simulink model "suivi_ligne_huit_eleve_2022b"  (R2024b)
settings: Solver=VariableStepAuto  StartTime=0.0  StopTime=140  RelTol=1e-3
InitFcn:
  | close all;
libraries: mobileRoboticsLib x2, visionsources x2, dspvision x2, visionsinks x2
settings Model: PacingRate=100  Creator=Caroline Lelandais  LastModifiedBy=radam
settings SolverCC: AlgebraicLoopSolver=TrustRegion
settings OptimizationCC: ReuseModelBlockBuffer=off
settings DebuggingCC: UnconnectedInputMsg=warning  UnconnectedOutputMsg=warning  UnconnectedLineMsg=warning
settings ModelReferenceCC: EnableRefExpFcnMdlSchedulingChecks=on
settings RTWCC: GPUComputeCapability=3.5

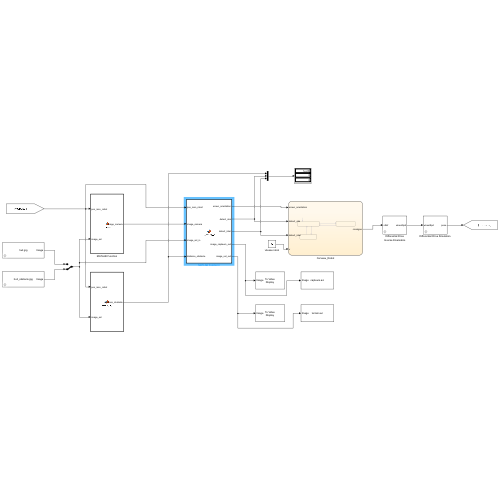
[thumbnail: Simulink's stored preview of the top-level diagram]
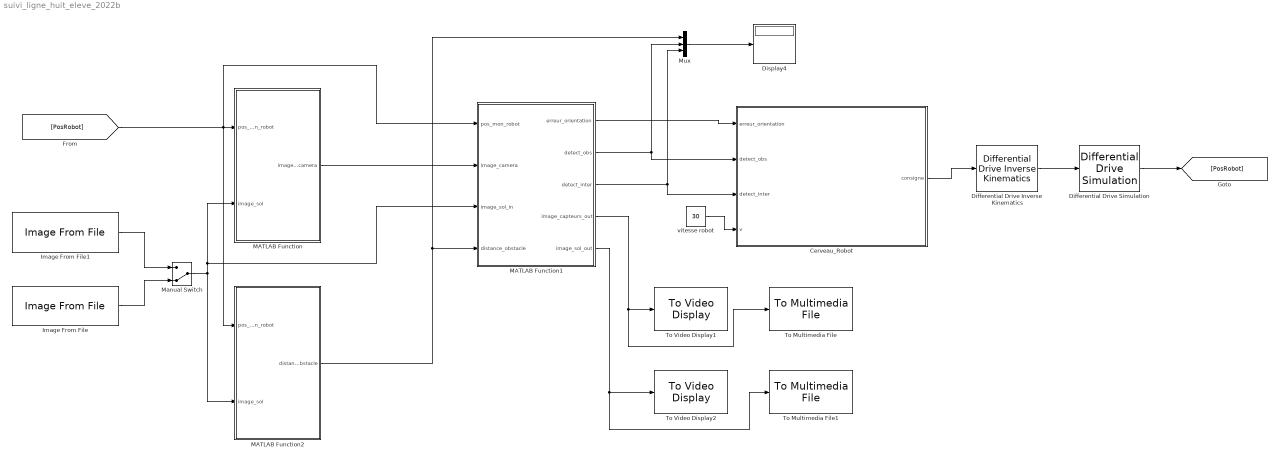
== system suivi_ligne_huit_eleve_2022b ==
  Cerveau_Robot : Stateflow chart  TreatAsAtomicUnit=on
  Differential Drive Inverse Kinematics : mobileRoboticsLib/Kinematic Models/Differential Drive/Differential Drive Inverse Kinematics  wheelRadius=0.1  wheelBase=0.5
      settings: SourceProductName=Mobile Robotics Simulation Toolbox
  Differential Drive Simulation : mobileRoboticsLib/Kinematic Models/Differential Drive/Differential Drive Simulation  wheelRadius=0.1  wheelBase=0.5  initX=291  initY=451  initAngle=2.4  Ts=0.1
      settings: SourceProductName=Mobile Robotics Simulation Toolbox
  Display4 : Display
  Image From File : visionsources/Image From File  Tag=vipblks_nd  FileName=huit_obstacle.jpg  Ts=inf  imagePorts=One multidimensional signal  OutPortLabels=R|G|B  ImageDataType=Inherit from input image  sdImageDataType=uint(8)  Signed=on  WordLength=16  FractionLengthMode=User-defined  FractionLength=15
  Image From File1 : visionsources/Image From File  Tag=vipblks_nd  FileName=huit.jpg  Ts=inf  imagePorts=One multidimensional signal  OutPortLabels=R|G|B  ImageDataType=Inherit from input image  sdImageDataType=uint(8)  Signed=on  WordLength=16  FractionLengthMode=User-defined  FractionLength=15
  MATLAB Function : MATLAB Function  TreatAsAtomicUnit=on
  MATLAB Function1 : MATLAB Function  TreatAsAtomicUnit=on
  MATLAB Function2 : MATLAB Function  TreatAsAtomicUnit=on
  Manual Switch : ManualSwitch  CurrentSetting=0
  Mux : Mux  Inputs=3
  To Multimedia File : dspvision/To Multimedia File  outputFilename=capteurs.avi  streamSelection=Video only  videoCompressor=None (uncompressed)  audioCompressor=None (uncompressed)  imagePorts=One multidimensional signal  fileType=AVI  audioDatatype=Determine from input data type  fourcc=RGB  audioBitRate=128  audioQuality=75  videoQuality=75  mj2000CompFactor=10
  To Multimedia File1 : dspvision/To Multimedia File  outputFilename=terrain.avi  streamSelection=Video only  videoCompressor=None (uncompressed)  audioCompressor=None (uncompressed)  imagePorts=One multidimensional signal  fileType=AVI  audioDatatype=Determine from input data type  fourcc=RGB  audioBitRate=128  audioQuality=75  videoQuality=75  mj2000CompFactor=10
  To Video Display1 : visionsinks/To Video Display  windowSizeMode=Normal  openAtMdlStart=on  fullScreen=off  videoWindowX=536805376  videoWindowY=536805376  saveWindowSize=off  videoWindowWidth=520  videoWindowHeight=352  inputColorFormat=RGB  inputType=Obsolete  imagePorts=One multidimensional signal  OutputDevice=On-screen video monitor  dataOrg=Column-major  isWindowOpen=off
  To Video Display2 : visionsinks/To Video Display  windowSizeMode=Normal  openAtMdlStart=on  fullScreen=off  videoWindowX=16  videoWindowY=88  saveWindowSize=off  videoWindowWidth=1247  videoWindowHeight=642  inputColorFormat=RGB  inputType=Obsolete  imagePorts=One multidimensional signal  OutputDevice=On-screen video monitor  dataOrg=Column-major  isWindowOpen=off
  vitesse robot : Constant  Value=30
  wires:
  Differential Drive Inverse Kinematics/1 -> Differential Drive Simulation/1
  Cerveau_Robot/1(consigne) -> Differential Drive Inverse Kinematics/1
  Differential Drive Simulation/1 -> [PosRobot]
  [PosRobot] -> MATLAB Function1/1(pos_mon_robot), MATLAB Function2/1(pos_mon_robot), MATLAB Function/1(pos_mon_robot)
  vitesse robot/1 -> Cerveau_Robot/4(v)
  MATLAB Function1/1(erreur_orientation) -> Cerveau_Robot/1(erreur_orientation)
  MATLAB Function1/2(detect_obs) -> Mux/2, Cerveau_Robot/2(detect_obs)
  MATLAB Function1/3(detect_inter) -> Mux/3, Cerveau_Robot/3(detect_inter)
  MATLAB Function1/4(image_capteurs_out) -> To Video Display1/1, To Multimedia File/1
  MATLAB Function1/5(image_sol_out) -> To Video Display2/1, To Multimedia File1/1
  MATLAB Function2/1(distance_obstacle) -> Mux/1, MATLAB Function1/4(distance_obstacle)
  MATLAB Function/1(image_camera) -> MATLAB Function1/2(image_camera)
  Manual Switch/1 -> MATLAB Function1/3(image_sol_in), MATLAB Function/2(image_sol), MATLAB Function2/2(image_sol)
  Image From File1/1 -> Manual Switch/1
  Image From File/1 -> Manual Switch/2
  Mux/1 -> Display4/1

== matlab function suivi_ligne_huit_eleve_2022b/MATLAB Function1 ==
  data: pos_mon_robot input; image_camera input; erreur_orientation output; detect_obs output; detect_inter output; image_sol_in input; image_capteurs_out output; image_sol_out output; distance_obstacle input
function [erreur_orientation, detect_obs, detect_inter, image_capteurs_out, image_sol_out] = Perception(pos_mon_robot, image_camera, image_sol_in, distance_obstacle)
%#codegen
% PERCEPTION (clean & simple, aligned with simplified Stateflow)
%   SuivreLigne : consigne = [v; erreur_orientation]
%   GererObs    : consigne = [0; +w_turn]  (handled in Stateflow)
%   GererInter  : consigne = [v; 0]        (handled in Stateflow)

% ---- init scalars ----
erreur_orientation = 0.0;  detect_obs = 0.0;  detect_inter = 0.0;

% ---- geometry ----
profondeur_camera=40; demi_largeur_camera=15;
profondeur_telemetre=80; demi_largeur_telemetre=5;
longueur_robot=30; demi_largeur_robot=10;

% ---- pose ----
px=round(pos_mon_robot(1)); py=round(pos_mon_robot(2)); th=pos_mon_robot(3);

% ---- memories ----
persistent ePrev obsLatch
if isempty(ePrev), ePrev=0; end
if isempty(obsLatch), obsLatch=0; end

% ---- outputs (fixed size) ----
image_capteurs_out=zeros(profondeur_telemetre,2*demi_largeur_camera,3,'uint8');
image_sol_out=image_sol_in; H=size(image_sol_out,1); W=size(image_sol_out,2);

% 1) LINE FOLLOWING — bottom 40% centroid on dark line
R=double(image_camera(:,:,1)); G=double(image_camera(:,:,2)); B=double(image_camera(:,:,3));
gray=0.2989*R+0.5870*G+0.1140*B;  Tdark=100;  isLine=(gray<Tdark);
rows=(profondeur_camera-round(0.4*profondeur_camera)+1):profondeur_camera; cols=1:(2*demi_largeur_camera);
colIdx=double(cols(:)); c0=demi_largeur_camera+0.5;
centers=nan(numel(rows),1);
for k=1:numel(rows)
    rr=rows(k); mask=isLine(rr,cols); n=nnz(mask);
    if n>0, centers(k)=sum(colIdx(mask))/n; end
end
Wrow=linspace(1,2,numel(rows))'; maskV=~isnan(centers);
cMean = c0; if any(maskV), cMean = sum(Wrow(maskV).*centers(maskV))/sum(Wrow(maskV)); end
offPix = c0 - cMean; offPix = max(-(demi_largeur_camera-3),min(demi_largeur_camera-3,offPix));
erreur_orientation = 0.6*ePrev + 0.4*offPix; ePrev=erreur_orientation;

% 2) OBSTACLE — simple distance with small hysteresis
dEnter=0.35*profondeur_telemetre; dExit=0.45*profondeur_telemetre;
d=double(distance_obstacle); if ~(isfinite(d))||d<=0||d>1e6, d=dExit+1; end
if obsLatch==0, if d<dEnter, obsLatch=1; end, else, if d>dExit, obsLatch=0; end, end
detect_obs=double(obsLatch);

% 3) INTERSECTION — white horizon test (only if no obstacle)
hRow=round(0.85*profondeur_camera); whiteCount=nnz(gray(hRow,:)>200);
detect_inter = double( (whiteCount/(2*demi_largeur_camera))>0.80 && detect_obs==0 );

% 4) VISUALS — same layout as before (camera, telemeter, overlays)
image_capteurs_out(1:profondeur_camera,1:2*demi_largeur_camera,:)=uint8(image_camera);
for i=(profondeur_camera+1):profondeur_telemetre
  for j=1:(2*demi_largeur_camera)
    c=(px+1j*py)+(i+1j*(j-demi_largeur_camera))*exp(1j*th);
    rr=min(max(1,round(real(c))),H); cc=min(max(1,round(imag(c))),W);
    image_capteurs_out(i,j,:)=image_sol_out(rr,cc,:);
  end
end
for i=1:longueur_robot
  for j=1:2*demi_largeur_robot
    c=(px+1j*py)-(i+1j*(j-demi_largeur_robot))*exp(1j*th);
    rr=min(max(1,round(real(c))),H); cc=min(max(1,round(imag(c))),W);
    image_sol_out(rr,cc,2)=255;
  end
end
for i=1:profondeur_camera
  for j=1:2*demi_largeur_camera
    c=(px+1j*py)+(i+1j*(j-demi_largeur_camera))*exp(1j*th);
    rr=min(max(1,round(real(c))),H); cc=min(max(1,round(imag(c))),W);
    image_sol_out(rr,cc,1)=255;
  end
end
for i=1:profondeur_telemetre
  for j=1:2*demi_largeur_telemetre
    c=(px+1j*py)+(i+1j*(j-demi_largeur_telemetre))*exp(1j*th);
    rr=min(max(1,round(real(c))),H); cc=min(max(1,round(imag(c))),W);
    image_sol_out(rr,cc,3)=255;
  end
end
pt=(px+1j*py)+(profondeur_camera/2+1j*erreur_orientation)*exp(1j*th);
r=min(max(1,round(real(pt))),H); c=min(max(1,round(imag(pt))),W);
image_sol_out(max(1,r-2):min(H,r+2),max(1,c-2):min(W,c+2),2)=255;
if abs(erreur_orientation)<(demi_largeur_camera-2)
  cc=round(demi_largeur_camera+0.5+erreur_orientation); lc=round(profondeur_camera/2);
  image_capteurs_out(max(1,lc-2):min(profondeur_camera,lc+2),max(1,cc-2):min(2*demi_largeur_camera,cc+2),2)=255;
end
image_capteurs_out(1,:,1)=240; image_capteurs_out(1:profondeur_camera,1,1)=240;
image_capteurs_out(profondeur_camera,:,1)=240; image_capteurs_out(1:profondeur_camera,end,1)=240;
k=(demi_largeur_camera-demi_largeur_telemetre);
image_capteurs_out(1,k:end-k,3)=240; image_capteurs_out(:,k,3)=240;
image_capteurs_out(end,k:end-k,3)=240; image_capteurs_out(:,end-k,3)=240;
image_capteurs_out=flipud(image_capteurs_out); image_capteurs_out=fliplr(image_capteurs_out);
image_sol_out(1:2,:,3)=240; image_sol_out(:,1:2,3)=240; image_sol_out(end-1:end,:,3)=240; image_sol_out(:,end-1:end,3)=240;
image_sol_out(px-1:px+1,py-1:py+1,2)=255;
end

== matlab function suivi_ligne_huit_eleve_2022b/MATLAB Function ==
  data: pos_mon_robot input; image_sol input; image_camera output
% Son rôle est de modéliser la photo brute prise par la caméra. Le modèle est extrêmement simplifié et fait comme si la photo était prise à la verticale et à l’avant du robot (par d’angle de vue).
% •	Entrées : pos_mon_robot (position du robot), image_sol (« terrain » soit la vue du ciel du circuit où doit évoluer le robot )
% •	Sorties : image_camera (vue du ciel du champ de vision du robot, rectangle rouge sur Video Display2)



function image_camera  = camera(pos_mon_robot, image_sol)

% Caractéristiques des coordonnées du champ de vision de la caméra 
profondeur_camera = 40;
demi_largeur_camera = 15;

% Récupération de la position du robot concerné
pos_x_vehicule = round(pos_mon_robot(1));
pos_y_vehicule = round(pos_mon_robot(2));
pos_angle_vehicule = pos_mon_robot(3);

%image vue par le capteur
image_camera=uint8(zeros(profondeur_camera,2*demi_largeur_camera,3));
for i=1:profondeur_camera
    for j=1:2*demi_largeur_camera
        c=(pos_x_vehicule+1j*pos_y_vehicule)+(i+1j*(j-demi_largeur_camera))*exp(1j*pos_angle_vehicule);
        image_camera(i,j,:)=image_sol(round(real(c)),round(imag(c)),:);
    end
end

== matlab function suivi_ligne_huit_eleve_2022b/MATLAB Function2 ==
  data: pos_mon_robot input; image_sol input; distance_obstacle output
% Son rôle est de modéliser le signal de sortie du télémètre à l’avant du robot.
% •	Entrées : pos_mon_robot (position du robot), image_sol (« terrain » soit la vue du ciel du circuit où doit évoluer le robot )
% •	Sorties : distance_obstacle (distance de l’obstacle)


function distance_obstacle    = telemetre(pos_mon_robot, image_sol)

% Caractéristiques des coordonnées du champ de vision du télémètre

profondeur_telemetre_x = 80;
largeur_telemetre_y = 5;

% Récupération de la position du robot concerné
pos_x_vehicule = round(pos_mon_robot(1));
pos_y_vehicule = round(pos_mon_robot(2));
pos_angle_vehicule = pos_mon_robot(3);

%image vue par le capteur et detection d'un obstacle
image_capteur2=uint8(zeros(profondeur_telemetre_x,2*largeur_telemetre_y,3));
distance_obstacle=100000;
for i=1:profondeur_telemetre_x
    for j=1:2*largeur_telemetre_y
        c=(pos_x_vehicule+1j*pos_y_vehicule)+(i+1j*(j-largeur_telemetre_y))*exp(1j*pos_angle_vehicule);
        image_capteur2(i,j,:)=image_sol(round(real(c)),round(imag(c)),:);
        if (image_capteur2(i,j,1)>200) && (image_capteur2(i,j,2)<50) && (image_capteur2(i,j,3)<50)   % obstacle simulé ici par couleur rouge
            distance_obstacle=min(distance_obstacle,abs((i+1j*j)-(0+1j*largeur_telemetre_y)));
        end
    end
end

== stateflow chart suivi_ligne_huit_eleve_2022b/Cerveau_Robot ==
  state SuivreLigne
    consigne = [v; erreur_orientation];
  state GererObs
    during: consigne=[0;+w]
  state GererInter
    during: consigne = [v; 0];
  (default) -> SuivreLigne
  SuivreLigne -> GererObs [order 1] : [detect_obs == 1]
  GererObs -> SuivreLigne : [after(pi/w, sec)]
  GererInter -> SuivreLigne : [after(2.5, sec)]
  SuivreLigne -> GererInter [order 2] : [detect_inter == 1 && detect_obs == 0]
  data: consigne output; erreur_orientation input; detect_obs input; detect_inter input; v input; w constant double =0.6
